simulink model "FeedbackControl"  (R2026a)
settings: Solver=FixedStepDiscrete  StopTime=15  FixedStep=0.01
undefined symbols (not defined in the file): g, ts_uav, UAVmass, waypoints
libraries: slpidlib x2
settings Model: DataDictionary=QuadData.sldd  Creator=The MathWorks, Inc.  LastModifiedBy=aylin.edgu
settings ModelReferenceCC: ModelReferenceNumInstancesAllowed=Single
settings RTWCC: SystemTargetFile=ert.tlc  GenerateMakefile=off  Description=Embedded Coder
settings ERTTargetCC: GenerateSampleERTMain=on

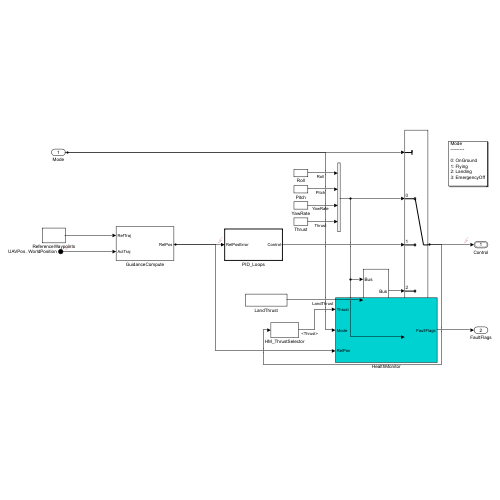
[thumbnail: Simulink's stored preview of the top-level diagram]
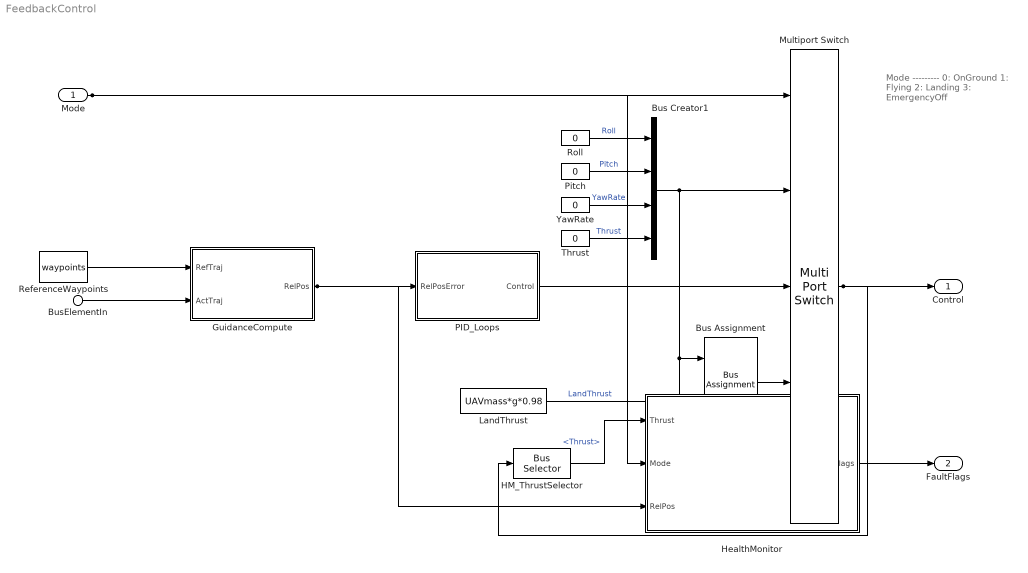
== system FeedbackControl ==
  note: Mode
      | ---------
      |
      | 0: OnGround
      | 1: Flying
      | 2: Landing
      | 3: EmergencyOff
  Mode : Inport  OutDataTypeStr=uint8  PortDimensions=1
  BusElementIn : Inport  Port=2  PortName=UAVPos  Element=WorldPosition
  Bus Assignment : BusAssignment  AssignedSignals=Thrust
  Bus Creator1 : BusCreator  Inputs=4  OutDataTypeStr=Bus: MultirotorGuidanceControlBus  NonVirtualBus=on
  GuidanceCompute : Subsystem
  HM_ThrustSelector : BusSelector  OutputSignals=Thrust
  HealthMonitor : Subsystem
  LandThrust : Constant  Value=UAVmass*g*0.98
  Multiport Switch : MultiPortSwitch  DataPortOrder=Zero-based contiguous  Inputs=4  zeroidx=on  SaturateOnIntegerOverflow=off  InputSameDT=off
  PID_Loops : Subsystem  TreatAsAtomicUnit=on
  Pitch : Constant  Value=0
  ReferenceWaypoints : Constant  Value=waypoints  SampleTime=ts_uav
  Roll : Constant  Value=0
  Thrust : Constant  Value=0
  YawRate : Constant  Value=0
  Control : Outport  OutDataTypeStr=Bus: MultirotorGuidanceControlBus
  FaultFlags : Outport  Port=2
  wires:
  Pitch/1 -> Bus Creator1/2  "Pitch"
  Bus Assignment/1 -> Multiport Switch/4
  PID_Loops/1(Control) -> Multiport Switch/3
  LandThrust/1 -> Bus Assignment/2  "LandThrust"
  Roll/1 -> Bus Creator1/1  "Roll"
  Bus Creator1/1 -> Multiport Switch/5, Bus Assignment/1, Multiport Switch/2
  Mode/1 -> Multiport Switch/1, HealthMonitor/2(Mode)
  Thrust/1 -> Bus Creator1/4  "Thrust"
  YawRate/1 -> Bus Creator1/3  "YawRate"
  Multiport Switch/1 -> Control/1, HM_ThrustSelector/1
  ReferenceWaypoints/1 -> GuidanceCompute/1(RefTraj)
  BusElementIn/1 -> GuidanceCompute/2(ActTraj)
  GuidanceCompute/1(RelPos) -> PID_Loops/1(RelPosError), HealthMonitor/3(RelPos)
  HM_ThrustSelector/1 -> HealthMonitor/1(Thrust)  "<Thrust>"
  HealthMonitor/1(FaultFlags) -> FaultFlags/1

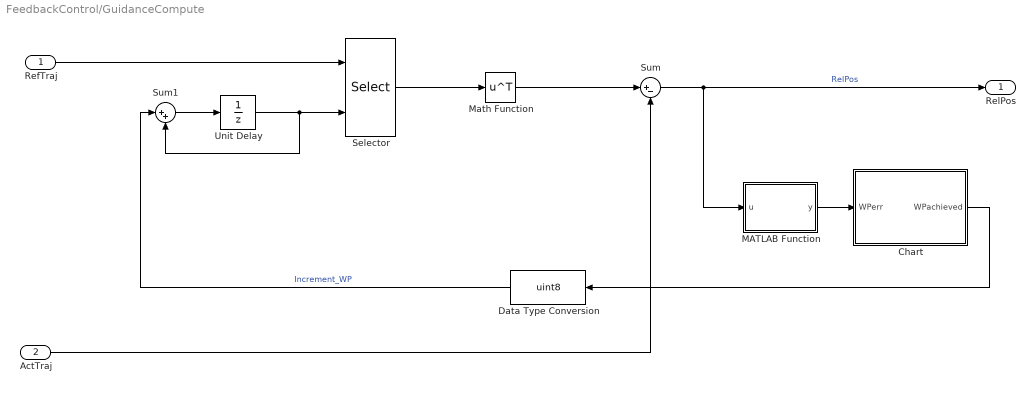
== system FeedbackControl/GuidanceCompute ==
  RefTraj : Inport
  ActTraj : Inport  Port=2
  Chart : Stateflow chart  TreatAsAtomicUnit=on
  Data Type Conversion : DataTypeConversion  OutDataTypeStr=uint8  SaturateOnIntegerOverflow=off  RndMeth=Floor
  MATLAB Function : MATLAB Function  TreatAsAtomicUnit=on
  Math Function : Math  Operator=transpose
  Selector : Selector  NumberOfDimensions=2  InputPortWidth=3  IndexOptions=Starting index (port),Select all  Indices=[1 3],1  OutputSizes=1,1
  Sum : Sum  Inputs=|+-
  Sum1 : Sum  Inputs=|++
  Unit Delay : UnitDelay  InitialCondition=1  SampleTime=-1
  RelPos : Outport
  wires:
  Unit Delay/1 -> Sum1/2, Selector/2
  Sum1/1 -> Unit Delay/1
  Math Function/1 -> Sum/1
  Sum/1 -> RelPos/1, MATLAB Function/1(u)  "RelPos"
  Data Type Conversion/1 -> Sum1/1  "Increment_WP"
  MATLAB Function/1(y) -> Chart/1(WPerr)
  Selector/1 -> Math Function/1
  Chart/1(WPachieved) -> Data Type Conversion/1
  ActTraj/1 -> Sum/2
  RefTraj/1 -> Selector/1

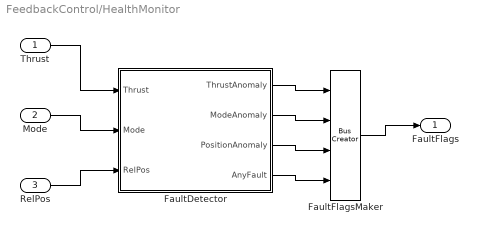
== system FeedbackControl/HealthMonitor ==
  Thrust : Inport
  Mode : Inport  Port=2
  RelPos : Inport  Port=3
  FaultDetector : MATLAB Function  TreatAsAtomicUnit=on
  FaultFlagsMaker : BusCreator  Inputs=4  OutDataTypeStr=Bus: FaultFlagsBus  NonVirtualBus=on
  FaultFlags : Outport
  wires:
  Thrust/1 -> FaultDetector/1(Thrust)
  Mode/1 -> FaultDetector/2(Mode)
  RelPos/1 -> FaultDetector/3(RelPos)
  FaultDetector/1(ThrustAnomaly) -> FaultFlagsMaker/1
  FaultDetector/2(ModeAnomaly) -> FaultFlagsMaker/2
  FaultDetector/3(PositionAnomaly) -> FaultFlagsMaker/3
  FaultDetector/4(AnyFault) -> FaultFlagsMaker/4
  FaultFlagsMaker/1 -> FaultFlags/1

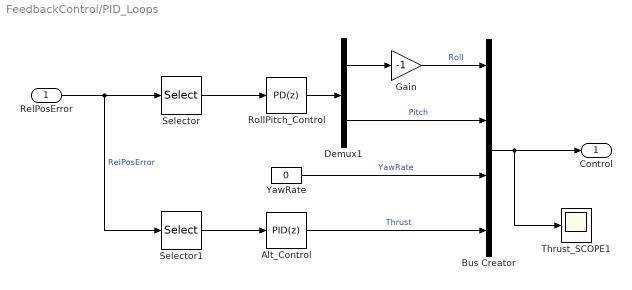
== system FeedbackControl/PID_Loops ==
  RelPosError : Inport
  Alt_Control : slpidlib/PID Controller  Controller=PID  Form=Parallel  TimeDomain=Discrete-time  UseExternalTs=off  SampleTime=ts_uav  IntegratorMethod=Forward Euler  FilterMethod=Forward Euler  ControllerParametersSource=internal  P=-0.213527398440291  I=-0.0449288545084318  UseKiTs=off  D=-0.253700825364154  UseExternalDerivativeSource=off  N=100  UseFilter=off  TunerSelectOption=Transfer Function Based (PID Tuner App)  InitialConditionSource=internal  InitialConditionForIntegrator=UAVmass*g  InitialConditionForFilter=0  DifferentiatorICPrevScaledInput=0  ExternalReset=none  TrackingMode=off  Kt=1  LimitOutput=off  SatLimitsSource=internal  UpperSaturationLimit=inf  LowerSaturationLimit=-inf  LinearizeAsGain=on  AntiWindupMode=none  Kb=1  LimitIntegrator=off  UpperIntegratorSaturationLimit=inf  LowerIntegratorSaturationLimit=-inf  POutMin=[]  POutMax=[]  IOutMin=[]  IOutMax=[]  DOutMin=[]  DOutMax=[]  NOutMin=[]  NOutMax=[]  SumOutMin=[]  SumOutMax=[]  SaturationOutMin=[]  SaturationOutMax=[]  PParamMin=[]  PParamMax=[]  IParamMin=[]  IParamMax=[]  DParamMin=[]  DParamMax=[]  NParamMin=[]  NParamMax=[]  KbParamMin=[]  KbParamMax=[]  KtParamMin=[]  KtParamMax=[]  KbOutMin=[]  KbOutMax=[]  KtOutMin=[]  KtOutMax=[]  IntegratorOutMin=[]  IntegratorOutMax=[]  FilterOutMin=[]  FilterOutMax=[]  SumI1OutMin=[]  SumI1OutMax=[]  SumI2OutMin=[]  SumI2OutMax=[]  SumI3OutMin=[]  SumI3OutMax=[]  SumI4OutMin=[]  SumI4OutMax=[]  SumDOutMin=[]  SumDOutMax=[]  DifferentiatorOutMin=[]  DifferentiatorOutMax=[]  FilterDiffOutCoefMin=[]  FilterDiffOutCoefMax=[]  ReciprocalOutMin=[]  ReciprocalOutMax=[]  SumDenOutMin=[]  SumDenOutMax=[]  SumNumOutMin=[]  SumNumOutMax=[]  DivideOutMin=[]  DivideOutMax=[]  UdiffTsProdOutMin=[]  UdiffTsProdOutMax=[]  NTsProdOutMin=[]  NTsProdOutMax=[]  UintegralTsProdOutMin=[]  UintegralTsProdOutMax=[]  UngainTsProdOutMin=[]  UngainTsProdOutMax=[]  ClampingZeroOutDataTypeStr=Inherit: Inherit via back propagation  ClampingZeroOutMin=[]  ClampingZeroOutMax=[]  FilterDenConstantOutDataTypeStr=Inherit: Inherit via back propagation  FilterDenConstantOutMin=[]  FilterDenConstantOutMax=[]  PCopyOutDataTypeStr=Inherit: Inherit via back propagation  PCopyOutMin=[]  PCopyOutMax=[]  NCopyOutDataTypeStr=Inherit: Inherit via back propagation  NCopyOutMin=[]  NCopyOutMax=[]  IntegratorContinuousStateAttributes=''  IntegratorStateMustResolveToSignalObject=off  IntegratorRTWStateStorageClass=Auto  FilterContinuousStateAttributes=''  FilterStateMustResolveToSignalObject=off  FilterRTWStateStorageClass=Auto  ParallelPVariant=InternalParameters  IdealPVariant=Disabled  IVariant=InternalParameters  DVariant=InternalParameters  IntegratorVariant=Discrete  SatVariant=Disabled  AWVariant=Passthrough  PCopyVariant=Disabled  TRVariant=Disabled  FdbkBlocksVariant=Forward  IdealPFdbkVariant=Disabled  SatFdbkVariant=Disabled  DerivativeFilterVariant=Differentiator  NVariant=Passthrough  NCopyVariant=Disabled_SignalSpec  FilterICVariant=InternalICsDifferentiator  IntegratorICVariant=InternalICs  ExternalResetVariant=Disabled  TRSumVariant=Passthrough  SumFdbkVariant=Disabled  SumVariant=Sum_PID  TsampFilterVariant=InternalTs  TsampNgainVariant=Passthrough  TsampIntegralVariant=Disabled_SignalSpec  ExternalSaturationOutDataTypeStr=Inherit: Same as second input  DerivativeSourceVariant=ErrorSignal  PreIntVariant=InternalPreInt
  Bus Creator : BusCreator  Inputs=4  OutDataTypeStr=Bus: MultirotorGuidanceControlBus  NonVirtualBus=on
  Demux1 : Demux  Outputs=2
  Gain : Gain  Gain=-1
  RollPitch_Control : slpidlib/PID Controller  Controller=PD  Form=Parallel  TimeDomain=Discrete-time  UseExternalTs=off  SampleTime=ts_uav  IntegratorMethod=Forward Euler  FilterMethod=Forward Euler  ControllerParametersSource=internal  P=-0.00720350415583028  I=1  UseKiTs=off  D=-0.205809687615586  UseExternalDerivativeSource=off  N=100  UseFilter=off  TunerSelectOption=Transfer Function Based (PID Tuner App)  InitialConditionSource=internal  InitialConditionForIntegrator=0  InitialConditionForFilter=0  DifferentiatorICPrevScaledInput=0  ExternalReset=none  TrackingMode=off  Kt=1  LimitOutput=off  SatLimitsSource=internal  UpperSaturationLimit=inf  LowerSaturationLimit=-inf  LinearizeAsGain=on  AntiWindupMode=none  Kb=1  LimitIntegrator=off  UpperIntegratorSaturationLimit=inf  LowerIntegratorSaturationLimit=-inf  POutMin=[]  POutMax=[]  IOutMin=[]  IOutMax=[]  DOutMin=[]  DOutMax=[]  NOutMin=[]  NOutMax=[]  SumOutMin=[]  SumOutMax=[]  SaturationOutMin=[]  SaturationOutMax=[]  PParamMin=[]  PParamMax=[]  IParamMin=[]  IParamMax=[]  DParamMin=[]  DParamMax=[]  NParamMin=[]  NParamMax=[]  KbParamMin=[]  KbParamMax=[]  KtParamMin=[]  KtParamMax=[]  KbOutMin=[]  KbOutMax=[]  KtOutMin=[]  KtOutMax=[]  IntegratorOutMin=[]  IntegratorOutMax=[]  FilterOutMin=[]  FilterOutMax=[]  SumI1OutMin=[]  SumI1OutMax=[]  SumI2OutMin=[]  SumI2OutMax=[]  SumI3OutMin=[]  SumI3OutMax=[]  SumI4OutMin=[]  SumI4OutMax=[]  SumDOutMin=[]  SumDOutMax=[]  DifferentiatorOutMin=[]  DifferentiatorOutMax=[]  FilterDiffOutCoefMin=[]  FilterDiffOutCoefMax=[]  ReciprocalOutMin=[]  ReciprocalOutMax=[]  SumDenOutMin=[]  SumDenOutMax=[]  SumNumOutMin=[]  SumNumOutMax=[]  DivideOutMin=[]  DivideOutMax=[]  UdiffTsProdOutMin=[]  UdiffTsProdOutMax=[]  NTsProdOutMin=[]  NTsProdOutMax=[]  UintegralTsProdOutMin=[]  UintegralTsProdOutMax=[]  UngainTsProdOutMin=[]  UngainTsProdOutMax=[]  ClampingZeroOutDataTypeStr=Inherit: Inherit via back propagation  ClampingZeroOutMin=[]  ClampingZeroOutMax=[]  FilterDenConstantOutDataTypeStr=Inherit: Inherit via back propagation  FilterDenConstantOutMin=[]  FilterDenConstantOutMax=[]  PCopyOutDataTypeStr=Inherit: Inherit via back propagation  PCopyOutMin=[]  PCopyOutMax=[]  NCopyOutDataTypeStr=Inherit: Inherit via back propagation  NCopyOutMin=[]  NCopyOutMax=[]  IntegratorContinuousStateAttributes=''  IntegratorStateMustResolveToSignalObject=off  IntegratorRTWStateStorageClass=Auto  FilterContinuousStateAttributes=''  FilterStateMustResolveToSignalObject=off  FilterRTWStateStorageClass=Auto  ParallelPVariant=InternalParameters  IdealPVariant=Disabled  IVariant=Disabled  DVariant=InternalParameters  IntegratorVariant=Disabled  SatVariant=Disabled  AWVariant=Disabled  PCopyVariant=Disabled  TRVariant=Disabled  FdbkBlocksVariant=Forward  IdealPFdbkVariant=Disabled  SatFdbkVariant=Disabled  DerivativeFilterVariant=Differentiator  NVariant=Passthrough  NCopyVariant=Disabled_SignalSpec  FilterICVariant=InternalICsDifferentiator  IntegratorICVariant=Disabled  ExternalResetVariant=Disabled  TRSumVariant=Passthrough  SumFdbkVariant=Disabled  SumVariant=Sum_PD  TsampFilterVariant=InternalTs  TsampNgainVariant=Passthrough  TsampIntegralVariant=Disabled_SignalSpec  ExternalSaturationOutDataTypeStr=Inherit: Same as second input  DerivativeSourceVariant=ErrorSignal  PreIntVariant=InternalPreInt
  Selector : Selector  InputPortWidth=3  IndexOptions=Index vector (dialog)  Indices=[2 1]  OutputSizes=1
  Selector1 : Selector  InputPortWidth=3  IndexOptions=Index vector (dialog)  Indices=3  OutputSizes=1
  Thrust_SCOPE1 : Scope
      settings: ActiveDisplayYMinimum=-0.12734  ActiveDisplayYMaximum=0.63082
  YawRate : Constant  Value=0
  Control : Outport
  wires:
  YawRate/1 -> Bus Creator/3  "YawRate"
  Alt_Control/1 -> Bus Creator/4  "Thrust"
  Bus Creator/1 -> Thrust_SCOPE1/1, Control/1
  RelPosError/1 -> Selector1/1, Selector/1  "RelPosError"
  RollPitch_Control/1 -> Demux1/1
  Selector/1 -> RollPitch_Control/1
  Demux1/1 -> Gain/1
  Demux1/2 -> Bus Creator/2  "Pitch"
  Selector1/1 -> Alt_Control/1
  Gain/1 -> Bus Creator/1  "Roll"

== matlab function FeedbackControl/HealthMonitor/FaultDetector ==
  data: Thrust input; ThrustAnomaly output; Mode input; RelPos input; ModeAnomaly output; PositionAnomaly output; AnyFault output
function [ThrustAnomaly, ModeAnomaly, PositionAnomaly, AnyFault] = detectFaults(Thrust, Mode, RelPos)
% HealthMonitor: detect anomalies in control, mode, and position signals
ThrustAnomaly   = Thrust < 0 || Thrust > 2.0;
ModeAnomaly     = Mode > uint8(3);
PositionAnomaly = any(isnan(RelPos)) || norm(double(RelPos)) > 10.0;
AnyFault        = ThrustAnomaly || ModeAnomaly || PositionAnomaly;
end

== matlab function FeedbackControl/GuidanceCompute/MATLAB Function ==
  data: u input; y output
function y = vector_norm(u)
    y = norm(u);
end

== stateflow chart FeedbackControl/GuidanceCompute/Chart ==
  state NotNearWP
    en: WPachieved = false;
  state NearWP
    en: count = 0; WPachieved = false;
    du: count = count+ts_uav;
  state WPachieved
    en: WPachieved = true;
  (default) -> NotNearWP
  NotNearWP -> NearWP : [WPerr <= 0.1]
  NearWP -> NotNearWP [order 1] : [WPerr > 0.1]
  WPachieved -> NotNearWP
  NearWP -> WPachieved [order 2] : [count >= 0.75]
  data: WPerr input; count local; WPachieved output; ts_uav parameter
